simulink model "chap6_5sim"  (Simulink 3.00)
settings: Solver=ode45  StartTime=0.0  StopTime=50  RelTol=1e-3
settings Model: LastModifiedBy=liu

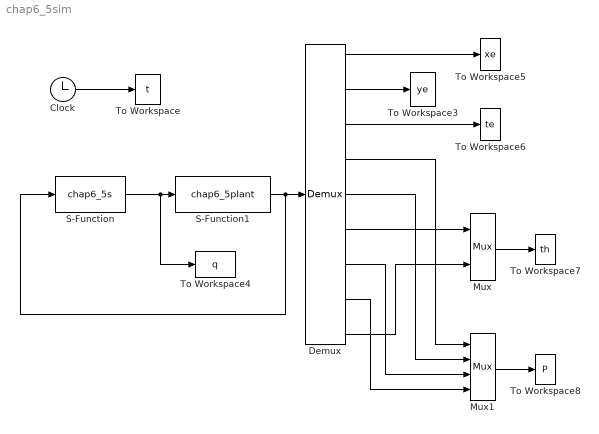
== system chap6_5sim ==
  Clock : Clock
      settings: DisplayTime=off  Decimation=10
  Demux : Demux  Outputs=9
  Mux : Mux  Inputs=2
      settings: DisplayOption=none
  Mux1 : Mux  Inputs=4
      settings: DisplayOption=none
  S-Function : S-Function  FunctionName=chap6_5s  PortCounts=[]  SFunctionModules=''
  S-Function1 : S-Function  FunctionName=chap6_5plant  PortCounts=[]  SFunctionModules=''
  To Workspace : ToWorkspace  VariableName=t  SampleTime=-1  SaveFormat=Matrix
  To Workspace3 : ToWorkspace  VariableName=ye  SampleTime=-1  SaveFormat=Matrix
  To Workspace4 : ToWorkspace  VariableName=q  SampleTime=-1  SaveFormat=Matrix
  To Workspace5 : ToWorkspace  VariableName=xe  SampleTime=-1  SaveFormat=Matrix
  To Workspace6 : ToWorkspace  VariableName=te  SampleTime=-1  SaveFormat=Matrix
  To Workspace7 : ToWorkspace  VariableName=th  SampleTime=-1  SaveFormat=Matrix
  To Workspace8 : ToWorkspace  VariableName=P  SampleTime=-1  SaveFormat=Matrix
  wires:
  S-Function1/1 -> Demux/1, S-Function/1
  S-Function/1 -> S-Function1/1, To Workspace4/1
  Demux/2 -> To Workspace3/1
  Demux/1 -> To Workspace5/1
  Demux/3 -> To Workspace6/1
  Mux/1 -> To Workspace7/1
  Demux/6 -> Mux/1
  Demux/9 -> Mux/2
  Clock/1 -> To Workspace/1
  Mux1/1 -> To Workspace8/1
  Demux/4 -> Mux1/1
  Demux/5 -> Mux1/2
  Demux/7 -> Mux1/3
  Demux/8 -> Mux1/4
